simulink model "ExponentialHornChoked_frequencyResponse"  (Simulink 7.8)
settings: Solver=FixedStepDiscrete  StartTime=0.0  StopTime=1.0  FixedStep=1.0  RelTol=1e-3
undefined symbols (not defined in the file): a_matrix, chokedExit, curvedDuct, d_matrix, x
settings Model: Creator=emmert  LastModifiedBy=smith

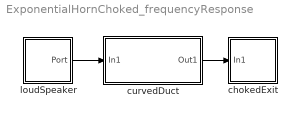
== system ExponentialHornChoked_frequencyResponse ==
  chokedExit : Subsystem  mask{Gamma=1.4}
      mask prompts: Gamma "Gamma (dimensionless)"
      mask Display:
      | patch([0 .6 .6 0],[.2 .2 .8 .8],[.7 1 1])
      | patch([.6 .7 .7 .6],[.2 .2 .8 .8],[.8 1 1])
      | patch([.7 .8 .8 .7],[.2 .2 .8 .8],[.9 1 1])
      | plot([0 .7 .7],[.2 .2 .35])
      | plot([0 .7 .7],[.8 .8 .65])
      | port_label('input',1,'M>1')
      | plot([1 1 0 0 1],[1 0 0 1 1])
  curvedDuct : Subsystem  mask{surface_poly=exp(2*x), d_Auto=on, d_polyin='1', l=1, n=25}
      mask prompts: surface_poly "Area function A(x) (m²)"; d_Auto "Diameter Automatic"; d_polyin "Diameter function D(x) (m)"; l "Lenght (m)"; n "Number of "discretization" elements"
      mask init:
      | mode=0;
      |    
      |    switch d_Auto
      |        case 1
      |            d_poly='-1';
      |        case 0 
      |            d_poly=d_polyin;   
      |    end
      |     
      |    tk=0;
      | 
      |    for kk = -0.5:1:n+1      
      |        tk=tk+1;
      |        xx=kk*l/n ;
      |        x=max(xx,0) ;
      |        x=min(x,l) ; 
      |        Di = double(eval(d_poly)); 
      |        switch d_Auto
      |            case 0
      |             if Di<0
      |               if mode~=0
      |                   errordlg('diameter must be positive','invalid diameter');
      |               else 
      |                errordlg('diameter must be bigger than or equal to zero','invalid diameter');
      |               end
      |             end
      |        
      |        if Di==0&&mode~=0
      |            errordlg('diameter must be positive','invalid diameter');
      |        end
      |        end    
      |        ai = double(eval(surface_poly));
      |        if ai<=0
      |            errordlg('areas must be positive','invalid areas');
      |        end
      |        d_matrix(tk,1)=Di;
      |        a_matrix(tk,1)=ai;
      |    end
      mask CallbackString:
      | |maskStr = get_param(gcb,'MaskValues');
      | 
      | % check if The checkbox is selected or not.
      | 
      | if strcmp(maskStr{2},'on')
      | 
      |     MaskVisibi=get_param(gcb,'MaskVisibilities');
      |     MaskVisibi{3}='off';
      |     set_param(gcb,'MaskVisibilities',MaskVisibi)
      | else
      |     MaskVisibi=get_param(gcb,'MaskVisibilities');
      |     MaskVisibi{3}='on';
      |     set_param(gcb,'MaskVisibilities',MaskVisibi)
      | end|||
      mask Display:
      | patch([0  .2 .3 .7 .8 1  1  .8 .7 .3 .2  0],...
      |       [.2 .1 .1 .3 .3 .2 .8 .7 .7 .9 .9 .8],[.7 1 1])
      | plot([0 .2 .3 .7 .8 1],[.2 .1 .1 .3 .3 .2])
      | plot([0 .2 .3 .7 .8 1],[.8 .9 .9 .7 .7 .8])
      | text(.4,.5,'A(x)','HorizontalAlignment','center')
      | plot([1 1 0 0 1],[1 0 0 1 1])
  loudSpeaker : Subsystem  mask{loc=Upstream, Amp=1, c=100, Mach=0, rho=1.2, D=1, element=loudSpeaker}
      mask prompts: loc "Location"; Amp "Foringamplitude [m/s]"; c "Speed of sound (m/s)"; Mach "Mach number (dimensionless)"; rho "Density (Kg/m³)"; D "Diameter (m)"
      mask init:
      | if Mach<0
      |    errordlg('Mach Number must be bigger than or equal to zero','invalid Mach Number');
      | end
      | 
      | 
      | if c<=0
      |     errordlg('speed of sound must be positive','invalid speed of sound');
      | end
      | 
      | 
      | if D<=0
      |      errordlg('diameter must be positive','invalid diameter');
      | 
      | end
      | 
      | 
      | if rho<=0
      |      errordlg('density must be positive','invalid density');
      | end
      | 
      | % Set identifier
      | set_param(gcb,'element',char('loudSpeaker'));
      | 
      | switchBCUpDownStream(gcb,loc);
      mask StyleString: popup(Downstream|Upstream),edit,edit,edit,edit,edit,edit
      mask Display:
      | plot([.2 .2 .4 .4 .2],[.6 .4 .4 .6 .6])
      | plot([.7 .7 .4 .4 .7],[.9 .1 .3 .7 .9])
  wires:
  loudSpeaker/1(Port) -> curvedDuct/1(In1)
  curvedDuct/1(Out1) -> chokedExit/1(In1)

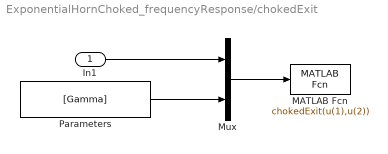
== system ExponentialHornChoked_frequencyResponse/chokedExit ==
  In1 : Inport
  MATLAB Fcn : MATLABFcn  MATLABFcn=chokedExit(u(1),u(2))  OutputDimensions=0
  Mux : Mux  Inputs=2
  Parameters : Constant  Value=[Gamma]
  wires:
  Parameters/1 -> Mux/2
  Mux/1 -> MATLAB Fcn/1
  In1/1 -> Mux/1

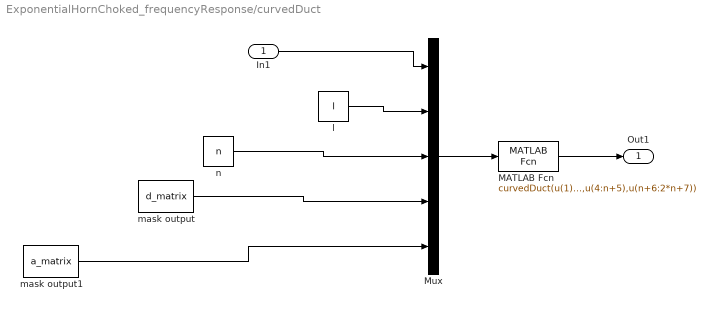
== system ExponentialHornChoked_frequencyResponse/curvedDuct ==
  In1 : Inport
  MATLAB Fcn : MATLABFcn  MATLABFcn=curvedDuct(u(1),u(2),u(3),u(4:n+5),u(n+6:2*n+7))  OutputDimensions=1
  Mux : Mux  Inputs=5
  l : Constant  Value=l
  mask output : Constant  Value=d_matrix
  mask output1 : Constant  Value=a_matrix
  n : Constant  Value=n
  Out1 : Outport
  wires:
  mask output1/1 -> Mux/5
  mask output/1 -> Mux/4
  n/1 -> Mux/3
  l/1 -> Mux/2
  MATLAB Fcn/1 -> Out1/1
  Mux/1 -> MATLAB Fcn/1
  In1/1 -> Mux/1

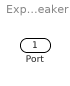
== system ExponentialHornChoked_frequencyResponse/loudSpeaker ==
  Port : Outport
